simulink model "observer_disturbance"  (R2017a)
settings: Solver=VariableStepAuto  StartTime=0.0  StopTime=0.5  RelTol=1e-3
values from neighbouring files (symbols this model uses):
  DCgain5 = D5d + C5cl*inv(eye(3)-A5cl)*B5d    [q13.m]    (also in q5.m; q5_reduced.m)
  h5 = 2.5*pi/w    [q13.m]    (also in q5.m = 2*pi/w; q5_reduced.m = 2*pi/w)
  K5_discr = place(A5d, B5d, P_discr)    [q13.m]    (also in q5.m; q5_reduced.m)
  L = place(A5d', C5d', P_discr6)    [q13.m]    (also in q5.m; q5_reduced.m)
  x0_obs = [0 0 0]    [q13.m]    (also in q5.m; q5_reduced.m)
  x0_plant = [-15 7 2]    [q13.m]    (also in q5.m; q5_reduced.m = [0.3 -0.5 0.1])
undefined symbols (not defined in the file or in its folder): A5d, B5d, C5d
settings Model: Creator=Aleksandra  LastModifiedBy=Aleksandra

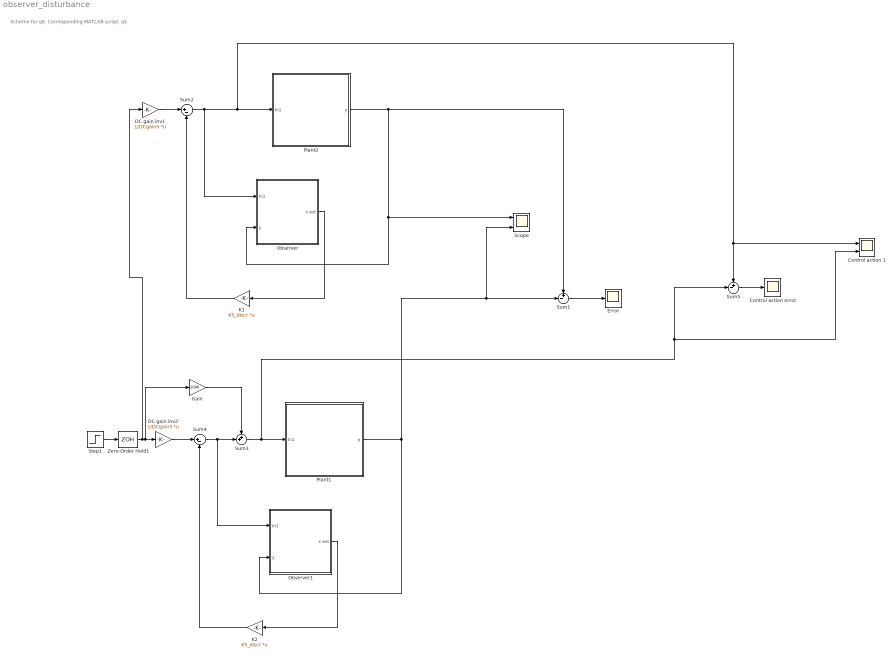
== system observer_disturbance ==
  note: Scheme for q6.
      | Corresponding MATLAB script: q5
  Control action 1 : Scope  NumInputPorts=2
  Control action error : Scope
  DC gain inv1 : Gain  Gain=1/DCgain5  Multiplication=Matrix(K*u)
  DC gain inv2 : Gain  Gain=1/DCgain5  Multiplication=Matrix(K*u)
  Error : Scope
  Gain : Gain  Gain=1000
  K1 : Gain  Gain=K5_discr  Multiplication=Matrix(K*u)
  K2 : Gain  Gain=K5_discr  Multiplication=Matrix(K*u)
  Observer : Subsystem
  Observer1 : Subsystem
  Plant1 : Subsystem
  Plant2 : Subsystem
  Scope : Scope  NumInputPorts=2
  Step1 : Step  Time=0  SampleTime=0
  Sum1 : Sum  Inputs=+-|
  Sum2 : Sum  Inputs=|+-
  Sum3 : Sum  Inputs=++|
  Sum4 : Sum  Inputs=|+-
  Sum5 : Sum  Inputs=+-|
  Zero-Order Hold1 : ZeroOrderHold  SampleTime=h5
  wires:
  K1/1 -> Sum2/2
  Observer/1(x est) -> K1/1
  DC gain inv1/1 -> Sum2/1
  Plant2/1(y) -> Sum1/1, Observer/2(y), Scope/1
  Step1/1 -> Zero-Order Hold1/1
  Zero-Order Hold1/1 -> DC gain inv1/1, Gain/1, DC gain inv2/1
  Sum4/1 -> Sum3/2, Observer1/1(In1)
  DC gain inv2/1 -> Sum4/1
  Observer1/1(x est) -> K2/1
  K2/1 -> Sum4/2
  Plant1/1(y) -> Scope/2, Sum1/2, Observer1/2(y)
  Sum1/1 -> Error/1
  Sum5/1 -> Control action error/1
  Sum2/1 -> Control action 1/1, Sum5/1, Plant2/1(In1), Observer/1(In1)
  Sum3/1 -> Control action 1/2, Sum5/2, Plant1/1(In1)
  Gain/1 -> Sum3/1

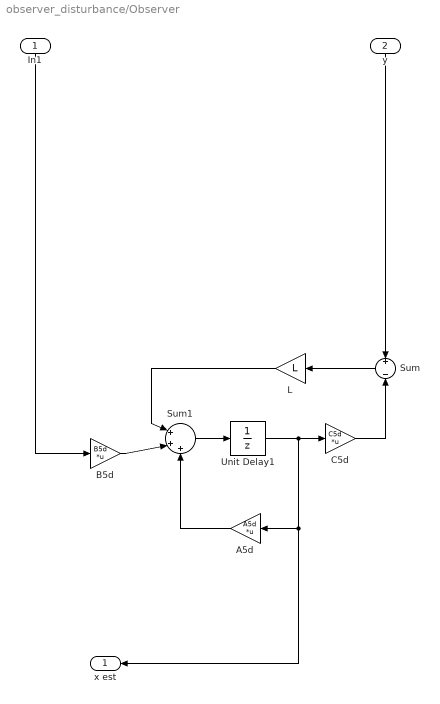
== system observer_disturbance/Observer ==
  In1 : Inport
  y : Inport  Port=2
  A5d : Gain  Gain=A5d  Multiplication=Matrix(K*u)
  B5d : Gain  Gain=B5d  Multiplication=Matrix(K*u)
  C5d : Gain  Gain=C5d  Multiplication=Matrix(K*u)
  L : Gain  Gain=L
  Sum : Sum  Inputs=+||-
  Sum1 : Sum  Inputs=|+++
  Unit Delay1 : UnitDelay  InitialCondition=x0_obs  SampleTime=-1
  x est : Outport
  wires:
  L/1 -> Sum1/1
  B5d/1 -> Sum1/2
  C5d/1 -> Sum/2
  A5d/1 -> Sum1/3
  Sum1/1 -> Unit Delay1/1
  In1/1 -> B5d/1
  y/1 -> Sum/1
  Unit Delay1/1 -> C5d/1, x est/1, A5d/1
  Sum/1 -> L/1

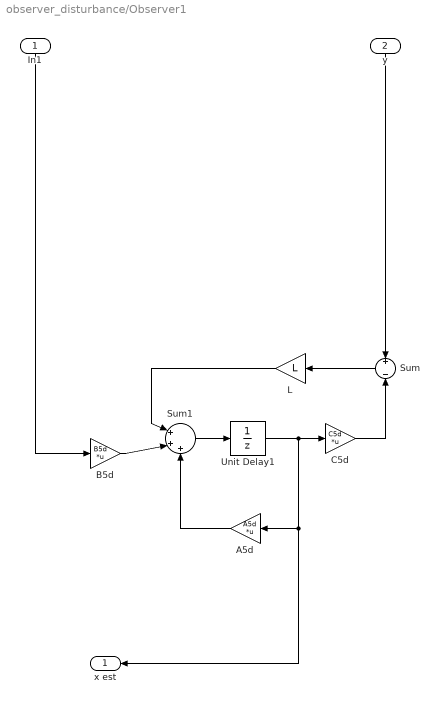
== system observer_disturbance/Observer1 ==
  In1 : Inport
  y : Inport  Port=2
  A5d : Gain  Gain=A5d  Multiplication=Matrix(K*u)
  B5d : Gain  Gain=B5d  Multiplication=Matrix(K*u)
  C5d : Gain  Gain=C5d  Multiplication=Matrix(K*u)
  L : Gain  Gain=L
  Sum : Sum  Inputs=+||-
  Sum1 : Sum  Inputs=|+++
  Unit Delay1 : UnitDelay  InitialCondition=x0_obs  SampleTime=-1
  x est : Outport
  wires:
  L/1 -> Sum1/1
  B5d/1 -> Sum1/2
  C5d/1 -> Sum/2
  A5d/1 -> Sum1/3
  Sum1/1 -> Unit Delay1/1
  In1/1 -> B5d/1
  y/1 -> Sum/1
  Unit Delay1/1 -> C5d/1, x est/1, A5d/1
  Sum/1 -> L/1

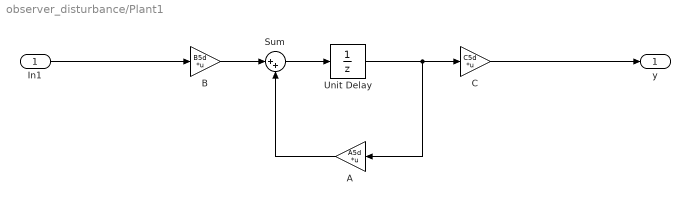
== system observer_disturbance/Plant1 ==
  In1 : Inport
  A : Gain  Gain=A5d  Multiplication=Matrix(K*u)
  B : Gain  Gain=B5d  Multiplication=Matrix(K*u)
  C : Gain  Gain=C5d  Multiplication=Matrix(K*u)
  Sum : Sum  Inputs=|++
  Unit Delay : UnitDelay  InitialCondition=x0_plant  SampleTime=-1
  y : Outport
  wires:
  Sum/1 -> Unit Delay/1
  A/1 -> Sum/2
  C/1 -> y/1
  B/1 -> Sum/1
  In1/1 -> B/1
  Unit Delay/1 -> A/1, C/1

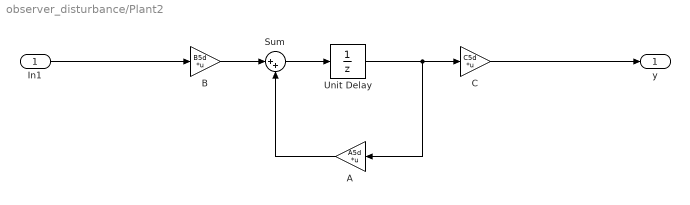
== system observer_disturbance/Plant2 ==
  In1 : Inport
  A : Gain  Gain=A5d  Multiplication=Matrix(K*u)
  B : Gain  Gain=B5d  Multiplication=Matrix(K*u)
  C : Gain  Gain=C5d  Multiplication=Matrix(K*u)
  Sum : Sum  Inputs=|++
  Unit Delay : UnitDelay  InitialCondition=x0_plant  SampleTime=-1
  y : Outport
  wires:
  Sum/1 -> Unit Delay/1
  A/1 -> Sum/2
  C/1 -> y/1
  B/1 -> Sum/1
  In1/1 -> B/1
  Unit Delay/1 -> A/1, C/1
